simulink model "quadrotorModel"  (R2020a)
settings: Solver=VariableStepAuto  StartTime=0.0  StopTime=10.0  RelTol=1e-3
undefined symbols (not defined in the file or in its folder): Ts, u0, x0
libraries: mympclib x1
settings Model: Creator=kohei  LastModifiedBy=kohei
settings DataIOCC: ReturnWorkspaceOutputs=off

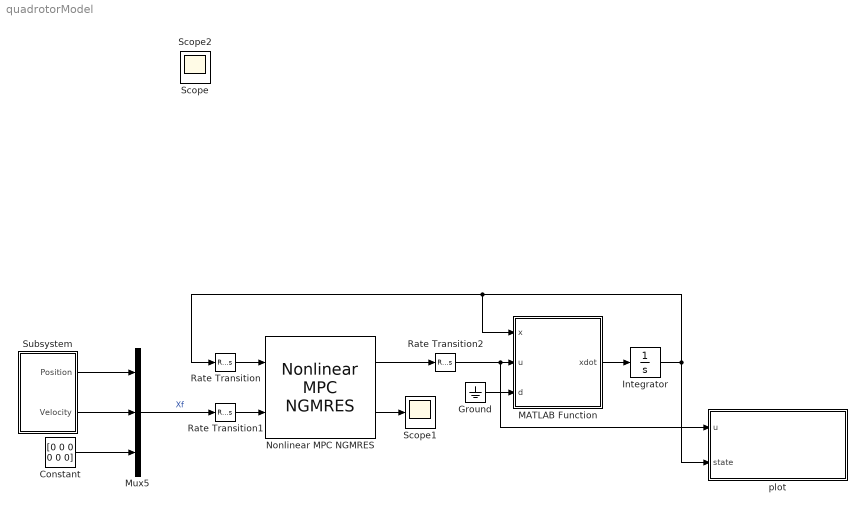
== system quadrotorModel ==
  Constant : Constant  Value=[0 0 0 0 0 0]
  Ground : Ground
  Integrator : Integrator  InitialCondition=x0
  MATLAB Function : MATLAB Function  TreatAsAtomicUnit=on
  Mux5 : Mux  Inputs=3
  Nonlinear MPC NGMRES : mympclib/Nonlinear MPC NGMRES  params=params  nx=12  nmv=4  ns=0  nL=0  Ts=Ts  enableDist=off  nd=1  enableYseq=off  enableFnorm=on
      settings: SourceProductName=My MPC Library
  Rate Transition : RateTransition  InitialCondition=x0
  Rate Transition1 : RateTransition
  Rate Transition2 : RateTransition  InitialCondition=u0(1:4)
  Scope1 : Scope
  Subsystem : Subsystem
  plot : Subsystem
  Scope : Scope
  Scope2 : Scope
  wires:
  Ground/1 -> MATLAB Function/3(d)
  MATLAB Function/1(xdot) -> Integrator/1
  Integrator/1 -> plot/2(state), MATLAB Function/1(x), Rate Transition/1
  Rate Transition/1 -> Nonlinear MPC NGMRES/1
  Rate Transition1/1 -> Nonlinear MPC NGMRES/2
  Rate Transition2/1 -> plot/1(u), MATLAB Function/2(u)
  Nonlinear MPC NGMRES/2 -> Scope1/1
  Nonlinear MPC NGMRES/1 -> Rate Transition2/1
  Mux5/1 -> Rate Transition1/1  "Xf"
  Subsystem/1(Position) -> Mux5/1
  Subsystem/2(Velocity) -> Mux5/2
  Constant/1 -> Mux5/3

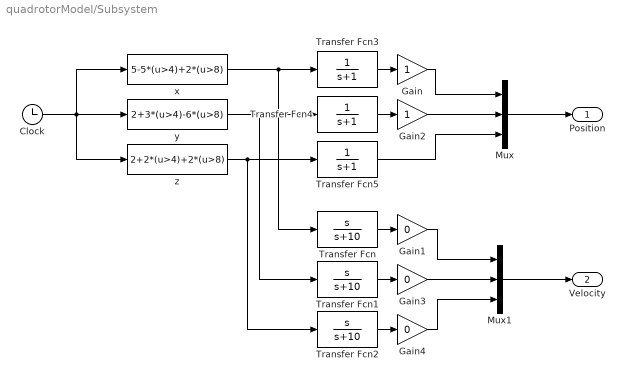
== system quadrotorModel/Subsystem ==
  Clock : Clock
  Gain : Gain
  Gain1 : Gain  Gain=0
  Gain2 : Gain
  Gain3 : Gain  Gain=0
  Gain4 : Gain  Gain=0
  Mux : Mux  Inputs=3
  Mux1 : Mux  Inputs=3
  Transfer Fcn : TransferFcn  Numerator=[1 0]  Denominator=[1 10]
  Transfer Fcn1 : TransferFcn  Numerator=[1 0]  Denominator=[1 10]
  Transfer Fcn2 : TransferFcn  Numerator=[1 0]  Denominator=[1 10]
  Transfer Fcn3 : TransferFcn  Denominator=[1 1]
  Transfer Fcn4 : TransferFcn  Denominator=[1 1]
  Transfer Fcn5 : TransferFcn  Denominator=[1 1]
  x : Fcn  Expr=5-5*(u>4)+2*(u>8)
  y : Fcn  Expr=2+3*(u>4)-6*(u>8)
  z : Fcn  Expr=2+2*(u>4)+2*(u>8)
  Position : Outport
  Velocity : Outport  Port=2
  wires:
  Clock/1 -> x/1, y/1, z/1
  x/1 -> Transfer Fcn/1, Transfer Fcn3/1
  y/1 -> Transfer Fcn1/1, Transfer Fcn4/1
  z/1 -> Transfer Fcn2/1, Transfer Fcn5/1
  Mux/1 -> Position/1
  Transfer Fcn/1 -> Gain1/1
  Transfer Fcn1/1 -> Gain3/1
  Transfer Fcn2/1 -> Gain4/1
  Mux1/1 -> Velocity/1
  Transfer Fcn3/1 -> Gain/1
  Transfer Fcn4/1 -> Gain2/1
  Transfer Fcn5/1 -> Mux/3
  Gain/1 -> Mux/1
  Gain1/1 -> Mux1/1
  Gain2/1 -> Mux/2
  Gain3/1 -> Mux1/2
  Gain4/1 -> Mux1/3

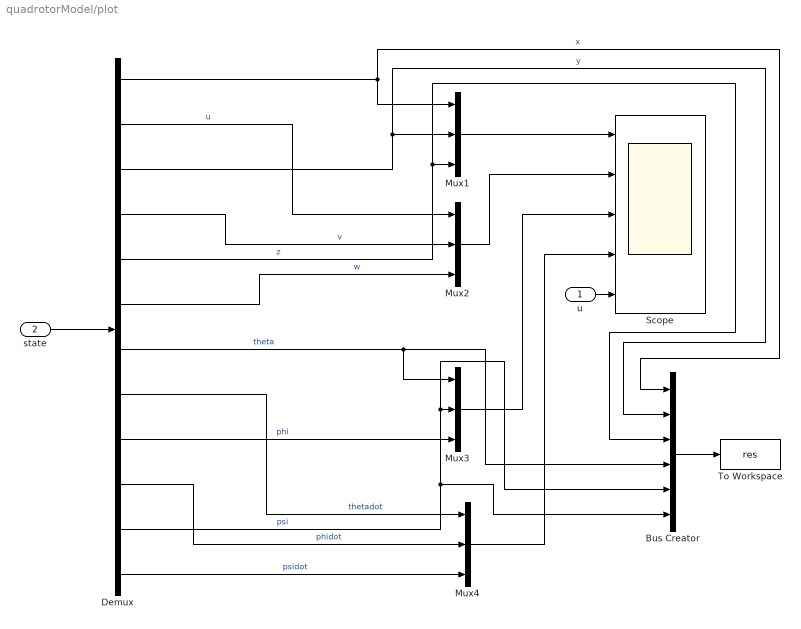
== system quadrotorModel/plot ==
  u : Inport
  state : Inport  Port=2
  Bus Creator : BusCreator  Inputs=6
  Demux : Demux  Outputs=12
  Mux{1..4} (4 alike) : Mux  Inputs=3
  Scope : Scope  NumInputPorts=5
  To Workspace : ToWorkspace  VariableName=res  SaveFormat=Timeseries  SampleTime=-1
  wires:
  u/1 -> Scope/5
  state/1 -> Demux/1
  Demux/4 -> Mux2/2  "v"
  Demux/6 -> Mux2/3  "w"
  Demux/1 -> Mux1/1, Bus Creator/1  "x"
  Mux1/1 -> Scope/1
  Demux/3 -> Mux1/2, Bus Creator/2  "y"
  Demux/2 -> Mux2/1  "u"
  Demux/5 -> Bus Creator/3, Mux1/3  "z"
  Mux2/1 -> Scope/2
  Mux3/1 -> Scope/3
  Bus Creator/1 -> To Workspace/1
  Demux/10 -> Mux4/2  "phidot"
  Demux/7 -> Mux3/1, Bus Creator/4  "theta"
  Mux4/1 -> Scope/4
  Demux/8 -> Mux4/1  "thetadot"
  Demux/9 -> Bus Creator/5, Mux3/2  "phi"
  Demux/11 -> Mux3/3, Bus Creator/6  "psi"
  Demux/12 -> Mux4/3  "psidot"

== matlab function quadrotorModel/MATLAB Function ==
  data: x input; u input; xdot output; d input
function xdot = fcn(x,u,d)
xdot = wrap_statefcn(x,u,d);
end
